simulink subsystem "DiffSwerveModuleSubsystem"  (R2022a)
settings: Solver=VariableStepAuto  StartTime=0.0  StopTime=10.0  RelTol=1e-3
values from neighbouring files (symbols this model uses):
  module = struct(     'M_inv', M_inv,     'J_w', J_w,     'Kt', Kt,     'Kv', Kv,     'Res', Res,     'sysc', sysc,     'sysd', sysd,     'lqr_K', lqr_K,     'Kff', Kff,     'D_w', D_w,     'Ts', Ts,     'Vmax', Vmax,     'Imax', Imax )    [GetDiffSwerveModule.m]    (also in RunDiffSwerveSimulation.m = GetDiffSwerveModule)
settings Model: Creator=woz4t  LastModifiedBy=woz4t

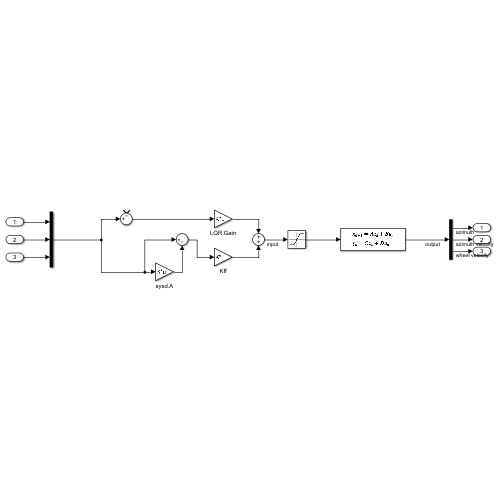
[thumbnail: Simulink's stored preview of the top-level diagram]
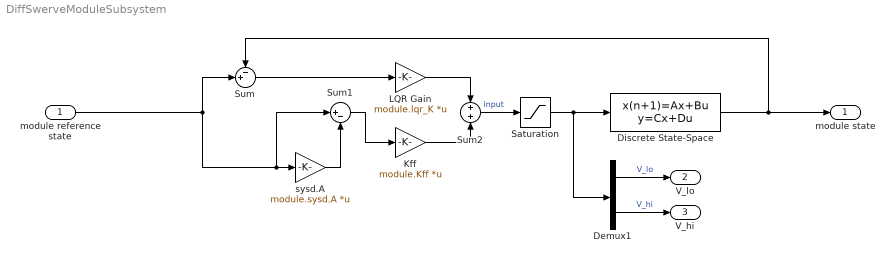
== system DiffSwerveModuleSubsystem ==
  module reference state : Inport
  Demux1 : Demux  Outputs=2
  Discrete State-Space : DiscreteStateSpace  A=module.sysd.A  B=module.sysd.B  C=module.sysd.C  D=module.sysd.D  SampleTime=module.Ts
  Kff : Gain  Gain=module.Kff  Multiplication=Matrix(K*u)
  LQR Gain : Gain  Gain=module.lqr_K  Multiplication=Matrix(K*u)
  Saturation : Saturate  UpperLimit=module.Vmax  LowerLimit=-module.Vmax
  Sum : Sum  Inputs=-+|
  Sum1 : Sum  Inputs=|+-
  Sum2 : Sum
  sysd.A : Gain  Gain=module.sysd.A  Multiplication=Matrix(K*u)
  module state : Outport
  V_lo : Outport  Port=2
  V_hi : Outport  Port=3
  wires:
  LQR Gain/1 -> Sum2/1
  Saturation/1 -> Discrete State-Space/1, Demux1/1
  Discrete State-Space/1 -> Sum/1, module state/1
  Sum/1 -> LQR Gain/1
  Sum1/1 -> Kff/1
  Kff/1 -> Sum2/2
  sysd.A/1 -> Sum1/2
  Sum2/1 -> Saturation/1  "input"
  module reference state/1 -> Sum/2, Sum1/1, sysd.A/1
  Demux1/2 -> V_hi/1  "V_hi"
  Demux1/1 -> V_lo/1  "V_lo"
